simulink model "RobotModel7"  (R2025b)
settings: Solver=VariableStepAuto  StartTime=0.0  StopTime=150  RelTol=0.01  AbsTol=0.01  EnableMultiTasking=on
undefined symbols (not defined in the file): waypoints, X, Y, Z
libraries: sm_lib x81, nesl_utility x35, slpidlib x2, robotalgslib x1, sharedtransform x1
(part 5 of 5)

== matlab function RobotModel7/RR_climb/MATLAB Function4 ==
  data: t input; q output; mode_cmd input
function q = knee_RL_motion(t, mode_cmd)
%#codegen
% --- 左后腿 (Rear Left) 膝关节 ---

% --- 时间节点 ---
T_squat_start = 102;
T_tuck_start  = 146;  % [新增] 开始收腿准备的时间（前腿搞定后）
T_climb_start = 155;  % 真正抬腿爬台阶的时间

% --- 阶段 0: 轮式 ---
if (mode_cmd == 1) || (t < T_squat_start)
    q = 0; return;
end

% ==========================================
% 阶段 1: 原地蹲起测试 (102s ~ 130s)
% ==========================================
if t < T_tuck_start
    tau = t - T_squat_start;
    q_stand = 0;
    q_squat = -deg2rad(70);
    T1 = 3; T2 = 15; T3 = 3;
    
    if tau < T1
        u = tau / T1;
        q = (1-u)*q_stand + u*q_squat;
    elseif tau < T1 + T2
        q = q_squat;
    elseif tau < T1 + T2 + T3
        u = (tau - (T1 + T2)) / T3;
        q = (1-u)*q_squat + u*q_stand;
    else
        q = q_stand;
    end
    return;
end

% ==========================================
% 阶段 2: [新增] 收腿预备 (Tuck) (130s ~ 153s)
% 核心策略：把后轮往前缩，缩短力臂，防止翻车
% ==========================================
q_stand = 0;
q_tuck  = deg2rad(-20);  % 收腿角度：膝盖弯曲40度，把轮子收进来

if t < T_climb_start
    tau = t - T_tuck_start;
    T_transition = 5.0; % 用5秒慢慢收腿，不要太快
    
    if tau < T_transition
        u = tau / T_transition;
        q = (1-u)*q_stand + u*q_tuck;
    else
        % 收完腿后保持住，等待起跳指令
        q = q_tuck; 
    end
    return;
end

% ==========================================
% 阶段 3: 爬台阶动作 (153s 开始)
% ==========================================
tau = t - T_climb_start;

% 爬台阶参数
% 注意：起始点现在是 q_tuck，不是 q_stand 了
q_lift  = deg2rad(-80); % 【重要】抬高：必须弯很多才能把轮子提上台阶
q_step  = deg2rad(-20);  % 落脚：上台阶后微屈

T_up   = 2.0;
T_hold = 3.0;
T_down = 2.0;

if tau < T_up
    % 1. 从收腿姿态 -> 抬起
    u = tau / T_up;
    q = (1-u)*q_tuck + u*q_lift; % 注意这里是从 q_tuck 开始变
    
elseif tau < (T_up + T_hold)
    % 2. 保持
    q = q_lift;
    
elseif tau < (T_up + T_hold + T_down)
    % 3. 放腿
    dt = tau - (T_up + T_hold);
    u = dt / T_down;
    q = (1-u)*q_lift + u*q_step;
    
else
    % 4. 保持在台阶上
    q = q_step;
end

end

== matlab function RobotModel7/RR/MATLAB Function ==
  data: mode_cmd input; alpha input; tau output; q input; dq input; q_cmd input; is_locked output; q_ref output
function [tau, is_locked, q_ref] = LockJointPD(mode_cmd, alpha, q, dq, q_cmd)
%#codegen
% mode_cmd: 0=Walk(folloew q_cmd), 1=Wheel(lock the present angle )
% alpha   : [0,1] flatten faktor(TransferFcnoutput)，0=walk, 1=leg locked
% q,dq    : joint angle/angular velocity
% q_cmd   : walking/standing angle(rad)

Kp = 1200.0;   % start value
Kd =   20.0;
tau_lim = 300.0;

m = uint8(mode_cmd ~= 0);     % uint8(0/1)
a = double(alpha);

persistent q_hold last_mode
if isempty(q_hold),    q_hold    = q;        end   % double
if isempty(last_mode), last_mode = uint8(0); end   % uint8

% step: 0->1 
if (last_mode == uint8(0)) && (m ~= uint8(0))
    q_hold = q;
end
last_mode = m;

% reference angle
q_ref  = a*q_hold + (1-a)*q_cmd;
dq_ref = 0.0;

% PD
tau = Kp*(q_ref - q) + Kd*(dq_ref - dq);

% 
tau = max(min(tau, tau_lim), -tau_lim);

% 
is_locked = (a > 0.5);     % 
end

== matlab function RobotModel7/RL/MATLAB Function4 ==
  data: t input; w output
function w = wheel_speed(t)

%#codegen

% --- 原始参数 ---

Tsw = 105; % 初次开始加速时间

Tacc = 2; % 加速时间 (0 -> V)

V = 100; % 力矩幅值 V

V2 = 20; % 力矩幅值 V2

Tdec_start = 125; % 开始减速 (V -> 0)

Tdec = 3; % 减速时间

Tpause = 5; % 停止后的等待时间

Treacc = 2; % 再次加速时间 (0 -> V2)

% --- 新增参数 (请根据需要调整数值) ---

Thold_V2 = 8; % V2 保持时间 (10秒)

Tdec2 = 3; % 第二次减速时间 (V2 -> 0) [假设为3秒]

Tpause2 = 10; % 第二次停止等待时间 (2秒)

Treacc2 = 2; % 第三次加速时间 (0 -> V2) [假设为2秒]

% --- 为了代码可读性，计算关键时间节点 ---

% 节点 1: V2 第一次加速完成的时间点 (即阶段 6 结束)

T_V2_ready = Tdec_start + Tdec + Tpause + Treacc;

% 节点 2: V2 保持 10秒 结束，开始减速的时间点

T_dec2_start = T_V2_ready + Thold_V2;

% 节点 3: 减速至 0 完成的时间点

T_stop2_start = T_dec2_start + Tdec2;

% 节点 4: 停止 2秒 结束，开始最后加速的时间点

T_last_acc_start = T_stop2_start + Tpause2;

% 节点 5: 最后加速至 V2 完成的时间点

T_final_stable = T_last_acc_start + Treacc2;

% ====================

% 逻辑判断

% ====================

% 阶段 1：未开始

if t < Tsw

w = 0;

% 阶段 2：线性加速 0 -> V

elseif t < Tsw + Tacc

u = (t - Tsw) / Tacc;

w = u * V;

% 阶段 3：保持 V

elseif t < Tdec_start

w = V;

% 阶段 4：线性减速 V -> 0

elseif t < Tdec_start + Tdec

u = (t - Tdec_start) / Tdec;

w = V * (1 - u);

% 阶段 5：停止等待

elseif t < Tdec_start + Tdec + Tpause

w = 0;

% 阶段 6：重新加速 0 -> V2

elseif t < T_V2_ready

u = (t - (Tdec_start + Tdec + Tpause)) / Treacc;

w = u * V2;

% --------------------

% 新增阶段开始

% --------------------

% 阶段 7：保持 V2 (10秒)

elseif t < T_dec2_start

w = V2;

% 阶段 8：再次减速 V2 -> 0

elseif t < T_stop2_start

u = (t - T_dec2_start) / Tdec2;

w = V2 * (1 - u);

% 阶段 9：再次停止等待 (2秒)

elseif t < T_last_acc_start

w = 0;

% 阶段 10：最后加速 0 -> V2

elseif t < T_final_stable

u = (t - T_last_acc_start) / Treacc2;

w = u * V2;

% 阶段 11：永久保持 V2

else

w = V2;

end

== matlab function RobotModel7/RR/MATLAB Function4 ==
  data: t input; w output
function w = wheel_speed(t)
%#codegen

Tsw  = 105;   % 初次开始加速时间
Tacc = 2;     % 加速时间
V    = 100;   % 力矩幅值
V2=18;

Tdec_start = 125;   % 开始减速
Tdec = 3;           % 减速时间
Tpause = 5;         % 停止后的等待时间
Treacc = 2;         % 再次加速时间

% --------------------
% 阶段 1：未开始
% --------------------
if t < Tsw
    w = 0;

% --------------------
% 阶段 2：线性加速 0→V
% --------------------
elseif t < Tsw + Tacc
    u = (t - Tsw) / Tacc;
    w = u * V;

% --------------------
% 阶段 3：保持 V
% --------------------
elseif t < Tdec_start
    w = V;

% --------------------
% 阶段 4：线性减速 V→0
% --------------------
elseif t < Tdec_start + Tdec
    u = (t - Tdec_start) / Tdec;  % 0→1
    w = V * (1 - u);

% --------------------
% 阶段 5：停止等待
% --------------------
elseif t < Tdec_start + Tdec + Tpause
    w = 0;

% --------------------
% 阶段 6：重新加速 0→V2
% --------------------
elseif t < Tdec_start + Tdec + Tpause + Treacc
    u = (t - (Tdec_start + Tdec + Tpause)) / Treacc;
    w = u * V2;

elseif t<Tdec_start + Tdec + Tpause + Treacc+3
    w=V2;
elseif t<Tdec_start + Tdec + Tpause + Treacc+3+2
    u=(t-(Tdec_start + Tdec + Tpause + Treacc+3))/2;
    w=u*V;
% --------------------
% 阶段 7：再次保持 V
% --------------------
else
    w = V;
end
end

== matlab function RobotModel7/FR/MATLAB Function ==
  data: mode_cmd input; alpha input; tau output; q input; dq input; q_cmd input; is_locked output; q_ref output
function [tau, is_locked, q_ref] = LockJointPD(mode_cmd, alpha, q, dq, q_cmd)
%#codegen
% mode_cmd: 0=Walk (track q_cmd), 1=Wheeled (lock current angle)
% alpha   : [0,1] smoothing factor (TransferFcn output), 0=fully walking, 1=fully locked
% q,dq    : joint angle/angular velocity
% q_cmd   : walk/stand target angle (radians)
Kp = 1200.0;   % Starting value, tune per joint
Kd =   20.0;
tau_lim = 300.0;
m = uint8(mode_cmd ~= 0);     % Standardize to uint8(0/1)
a = double(alpha);
persistent q_hold last_mode
if isempty(q_hold),    q_hold    = q;        end   % double
if isempty(last_mode), last_mode = uint8(0); end   % uint8
% Rising edge: 0->1, latch current angle
if (last_mode == uint8(0)) && (m ~= uint8(0))
    q_hold = q;
end
last_mode = m;
% Reference angle: interpolate between "hold angle" and "target angle"
q_ref  = a*q_hold + (1-a)*q_cmd;
dq_ref = 0.0;
% PD
tau = Kp*(q_ref - q) + Kd*(dq_ref - dq);
% Saturation
tau = max(min(tau, tau_lim), -tau_lim);
% Debug flag: is leg lock dominant
is_locked = (a > 0.5);     % Can also output m==1
end

== matlab function RobotModel7/FR/MATLAB Function1 ==
  data: mode_cmd input; alpha input; tau output; q input; dq input; q_cmd input; is_locked output; q_ref output
function [tau, is_locked, q_ref] = LockJointPD(mode_cmd, alpha, q, dq, q_cmd)
%#codegen
% mode_cmd: 0=Walk (track q_cmd), 1=Wheeled (lock current angle)
% alpha   : [0,1] smoothing factor (TransferFcn output), 0=fully walking, 1=fully locked
% q,dq    : joint angle/angular velocity
% q_cmd   : walk/stand target angle (radians)
Kp = 1200.0;   % Starting value, tune per joint
Kd =   20.0;
tau_lim = 300.0;
m = uint8(mode_cmd ~= 0);     % Standardize to uint8(0/1)
a = double(alpha);
persistent q_hold last_mode
if isempty(q_hold),    q_hold    = q;        end   % double
if isempty(last_mode), last_mode = uint8(0); end   % uint8
% Rising edge: 0->1, latch current angle
if (last_mode == uint8(0)) && (m ~= uint8(0))
    q_hold = q;
end
last_mode = m;
% Reference angle: interpolate between "hold angle" and "target angle"
q_ref  = a*q_hold + (1-a)*q_cmd;
dq_ref = 0.0;
% PD
tau = Kp*(q_ref - q) + Kd*(dq_ref - dq);
% Saturation
tau = max(min(tau, tau_lim), -tau_lim);
% Debug flag: is leg lock dominant
is_locked = (a > 0.5);     % Can also output m==1
end

== matlab function RobotModel7/FL/MATLAB Function ==
  data: mode_cmd input; alpha input; tau output; q input; dq input; q_cmd input; is_locked output; q_ref output
function [tau, is_locked, q_ref] = LockJointPD(mode_cmd, alpha, q, dq, q_cmd)
%#codegen
% mode_cmd: 0=Walk (track q_cmd), 1=Wheeled (lock current angle)
% alpha   : [0,1] smoothing factor (TransferFcn output), 0=fully walking, 1=fully locked
% q,dq    : joint angle/angular velocity
% q_cmd   : walk/stand target angle (radians)
Kp = 1200.0;   % Starting value, tune per joint
Kd =   20.0;
tau_lim = 300.0;
m = uint8(mode_cmd ~= 0);     % Standardize to uint8(0/1)
a = double(alpha);
persistent q_hold last_mode
if isempty(q_hold),    q_hold    = q;        end   % double
if isempty(last_mode), last_mode = uint8(0); end   % uint8
% Rising edge: 0->1, latch current angle
if (last_mode == uint8(0)) && (m ~= uint8(0))
    q_hold = q;
end
last_mode = m;
% Reference angle: interpolate between "hold angle" and "target angle"
q_ref  = a*q_hold + (1-a)*q_cmd;
dq_ref = 0.0;
% PD
tau = Kp*(q_ref - q) + Kd*(dq_ref - dq);
% Saturation
tau = max(min(tau, tau_lim), -tau_lim);
% Debug flag: is leg lock dominant
is_locked = (a > 0.5);     % Can also output m==1
end

== matlab function RobotModel7/FL/MATLAB Function1 ==
  data: mode_cmd input; alpha input; tau output; q input; dq input; q_cmd input; is_locked output; q_ref output
function [tau, is_locked, q_ref] = LockJointPD(mode_cmd, alpha, q, dq, q_cmd)
%#codegen
% mode_cmd: 0=Walk (track q_cmd), 1=Wheeled (lock current angle)
% alpha   : [0,1] smoothing factor (TransferFcn output), 0=fully walking, 1=fully locked
% q,dq    : joint angle/angular velocity
% q_cmd   : walk/stand target angle (radians)
Kp = 1200.0;   % Starting value, tune per joint
Kd =   20.0;
tau_lim = 300.0;
m = uint8(mode_cmd ~= 0);     % Standardize to uint8(0/1)
a = double(alpha);
persistent q_hold last_mode
if isempty(q_hold),    q_hold    = q;        end   % double
if isempty(last_mode), last_mode = uint8(0); end   % uint8
% Rising edge: 0->1, latch current angle
if (last_mode == uint8(0)) && (m ~= uint8(0))
    q_hold = q;
end
last_mode = m;
% Reference angle: interpolate between "hold angle" and "target angle"
q_ref  = a*q_hold + (1-a)*q_cmd;
dq_ref = 0.0;
% PD
tau = Kp*(q_ref - q) + Kd*(dq_ref - dq);
% Saturation
tau = max(min(tau, tau_lim), -tau_lim);
% Debug flag: is leg lock dominant
is_locked = (a > 0.5);     % Can also output m==1
end

== matlab function RobotModel7/RL/MATLAB Function ==
  data: mode_cmd input; alpha input; tau output; q input; dq input; q_cmd input; is_locked output; q_ref output
function [tau, is_locked, q_ref] = LockJointPD(mode_cmd, alpha, q, dq, q_cmd)
%#codegen
% mode_cmd: 0=Walk (track q_cmd), 1=Wheeled (lock current angle)
% alpha   : [0,1] smoothing factor (TransferFcn output), 0=fully walking, 1=fully locked
% q,dq    : joint angle/angular velocity
% q_cmd   : walk/stand target angle (radians)
Kp = 1200.0;   % Starting value, tune per joint
Kd =   20.0;
tau_lim = 300.0;
m = uint8(mode_cmd ~= 0);     % Standardize to uint8(0/1)
a = double(alpha);
persistent q_hold last_mode
if isempty(q_hold),    q_hold    = q;        end   % double
if isempty(last_mode), last_mode = uint8(0); end   % uint8
% Rising edge: 0->1, latch current angle
if (last_mode == uint8(0)) && (m ~= uint8(0))
    q_hold = q;
end
last_mode = m;
% Reference angle: interpolate between "hold angle" and "target angle"
q_ref  = a*q_hold + (1-a)*q_cmd;
dq_ref = 0.0;
% PD
tau = Kp*(q_ref - q) + Kd*(dq_ref - dq);
% Saturation
tau = max(min(tau, tau_lim), -tau_lim);
% Debug flag: is leg lock dominant
is_locked = (a > 0.5);     % Can also output m==1
end
